simulink model "hbridgeonlylinear"  (R2013b)
settings: Solver=FixedStepDiscrete  SolverMode=SingleTasking  StartTime=0.0  StopTime=inf  RelTol=1e-3
libraries: arduinolib x6
settings Model: SimulationMode=external  ExtModeTrigDuration=2  Creator=Joshua  LastModifiedBy=Joshua
settings OptimizationCC: OptimizeModelRefInitCode=on  LifeSpan=1
settings DebuggingCC: SolverPrmCheckMsg=none
settings HardwareCC: ProdBitPerInt=16  ProdBitPerPointer=8  ProdIntDivRoundTo=Zero  ProdEndianess=LittleEndian  ProdWordSize=8  ProdHWDeviceType=Atmel->AVR
settings RTWCC: SystemTargetFile=realtime.tlc  GenerateMakefile=off  TemplateMakefile=realtime.tmf  Description=Run on Target Hardware  RTWVerbose=off  ProcessScript=realtime_make_rtw_hook
settings STFCustomTargetCC: TargetLibSuffix=.a  GenerateSampleERTMain=on  ERTCustomFileBanners=on  SupportNonInlinedSFcns=off  SupportVariableSizeSignals=on  MATLABClassNameForMDSCustomization=Simulink.SoftwareTarget.ERTCustomization  GRTInterface=off  SystemTargetFile=realtime.tlc
settings ERTTargetCC: CodeReplacementLibrary=ANSI_C  GenerateSampleERTMain=on  ParMdlRefBuildCompliant=off  CompOptLevelCompliant=off  ConcurrentExecutionCompliant=off  CombineOutputUpdateFcns=off  ERTFirstTimeCompliant=off  SupportContinuousTime=on  SupportVariableSizeSignals=on  ModelStepFunctionPrototypeControlCompliant=off  CPPClassGenCompliant=off  ExtModeTransport=3  ExtModeMexFile=ext_serial_win32_comm  ExtModeMexArgs=0 1 9600  InlinedParameterPlacement=NonHierarchical  ERTSrcFileBannerTemplate=realtime_code_template.cgt  ERTHdrFileBannerTemplate=realtime_code_template.cgt  ERTDataSrcFileTemplate=realtime_code_template.cgt  ERTDataHdrFileTemplate=realtime_code_template.cgt  ERTCustomFileTemplate=realtime_file_process.tlc

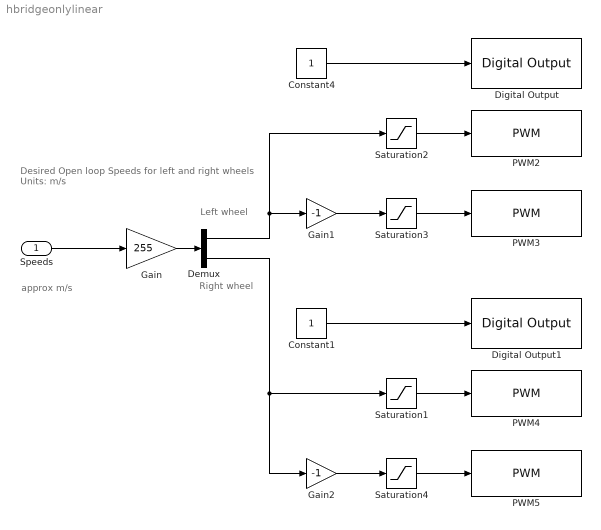
== system hbridgeonlylinear ==
  note: Right wheel
  note: Left wheel
  note: approx m/s
  note: Desired Open loop Speeds for left and right wheels
      | Units: m/s
  Speeds : Inport
  Constant1 : Constant
  Constant4 : Constant
  Demux : Demux  Outputs=2
  Digital Output : arduinolib/Digital Output  pinNumber=8
  Digital Output1 : arduinolib/Digital Output  pinNumber=13
  Gain : Gain  Gain=255
  Gain1 : Gain  Gain=-1
  Gain2 : Gain  Gain=-1
  PWM2 : arduinolib/PWM  pinNumber=9
  PWM3 : arduinolib/PWM  pinNumber=10
  PWM4 : arduinolib/PWM  pinNumber=11
  PWM5 : arduinolib/PWM  pinNumber=12
  Saturation{1..4} (4 alike) : Saturate  UpperLimit=255  LowerLimit=0  OutDataTypeStr=uint8
  wires:
  Speeds/1 -> Gain/1
  Gain/1 -> Demux/1
  Constant1/1 -> Digital Output1/1
  Demux/1 -> Saturation2/1, Gain1/1
  Constant4/1 -> Digital Output/1
  Saturation2/1 -> PWM2/1
  Saturation3/1 -> PWM3/1
  Gain1/1 -> Saturation3/1
  Demux/2 -> Gain2/1, Saturation1/1
  Gain2/1 -> Saturation4/1
  Saturation1/1 -> PWM4/1
  Saturation4/1 -> PWM5/1
